simulink model "AAIR4"  (R2020a)
settings: Solver=FixedStepAuto  StartTime=0.0  StopTime=10.0  FixedStep=1e-3  RelTol=1e-3  EnableMultiTasking=on
undefined symbols (not defined in the file): D0, D10, D11, D13, D2, D4, D5, D6, D8, PTA0, PTA2, PTB23, PTB9, PTC16, PTC2, PTD0, PTD1, PTD2
libraries: frdmk64flib x15, dspstat3 x1
settings Model: ExtModeTrigDuration=5  Creator=guga  LastModifiedBy=guga
settings OptimizationCC: EnhancedBackFolding=on  PassReuseOutputArgsAs=Individual arguments  ZeroExternalMemoryAtStartup=off  ZeroInternalMemoryAtStartup=off  MaxStackSize=64  OptimizeBlockOrder=speed  DifferentSizesBufferReuse=on  OptimizationCustomize=off  EfficientTunableParamExpr=on
settings DebuggingCC: ParameterTunabilityLossMsg=error
settings HardwareCC: ProdBitPerPointer=32  ProdBitPerSizeT=32  ProdBitPerPtrDiffT=32  ProdLargestAtomicInteger=Long  ProdLargestAtomicFloat=Double  ProdWordSize=32  ProdHWDeviceType=ARM Compatible->ARM Cortex
settings SFSimCC: MATLABDynamicMemAlloc=off
settings RTWCC: SystemTargetFile=ert.tlc  HardwareBoard=NXP FRDM-K64F  TemplateMakefile=ert_default_tmf  Toolchain=GNU Tools for ARM Embedded Processors
settings CodeAppCC: ForceParamTrailComments=on  IgnoreCustomStorageClasses=off  OperatorAnnotations=on  SimulinkDataObjDesc=on  SFDataObjDesc=on  InsertBlockDesc=on

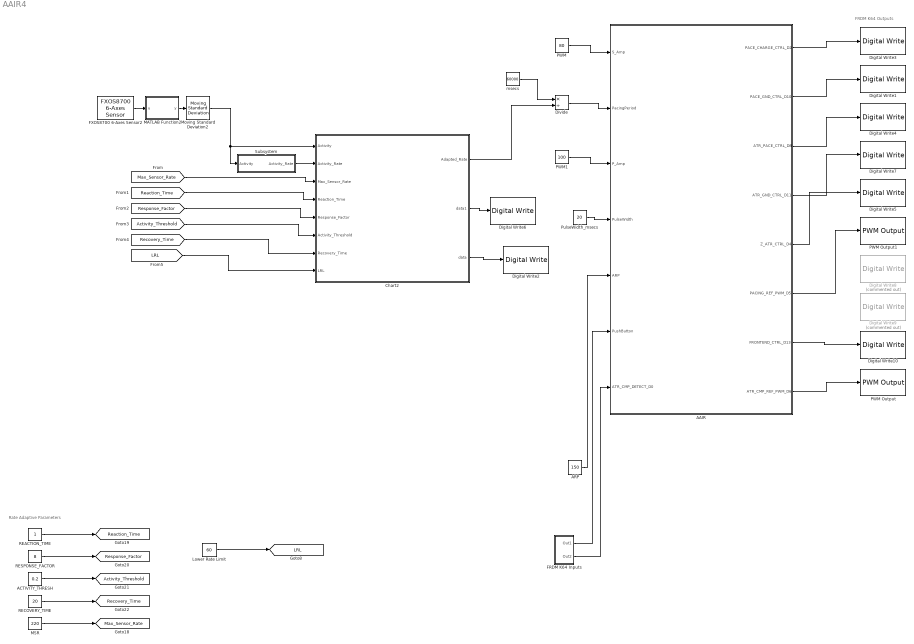
== system AAIR4 ==
  note: FRDM K64 Outputs
  note: Rate Adaptive Parameters
  AAIR : Stateflow chart  TreatAsAtomicUnit=on
  ACTIVITY_THRESH : Constant  Value=0.2  OutDataTypeStr=double
  ARP : Constant  Value=150
  Chart2 : Stateflow chart  TreatAsAtomicUnit=on
  Digital Write1 : frdmk64flib/Digital Write  Whichpin=PTD0 (D10)
  Digital Write10 : frdmk64flib/Digital Write  Whichpin=PTD1 (D13)
  Digital Write2 : frdmk64flib/Digital Write  Whichpin=RED_LED
  Digital Write3 : frdmk64flib/Digital Write  Whichpin=PTB9 (D2)
  Digital Write4 : frdmk64flib/Digital Write  Whichpin=PTA0 (D8)
  Digital Write5 : frdmk64flib/Digital Write  Whichpin=PTB23 (D4)
  Digital Write6 : frdmk64flib/Digital Write  Whichpin=GREEN_LED
  Digital Write7 : frdmk64flib/Digital Write  Whichpin=PTD2 (D11)
  Digital Write8 : frdmk64flib/Digital Write  Commented=on  Whichpin=RED_LED
  Digital Write9 : frdmk64flib/Digital Write  Commented=on  Whichpin=GREEN_LED
  Divide : Product  Inputs=*/
  FRDM K64 Inputs : Subsystem
  FXOS8700 6-Axes Sensor2 : frdmk64flib/FXOS8700 6-Axes Sensor  Activesensor=Accelerometer only  ODR=100Hz  HybridODR=400Hz  Accelfullrange=-4g to +4g  SampleTime=1/100
  Lower Rate Limit : Constant  Value=60  OutDataTypeStr=uint16
  MATLAB Function2 : MATLAB Function  TreatAsAtomicUnit=on
  MSR : Constant  Value=220  OutDataTypeStr=uint16
  Moving Standard Deviation2 : dspstat3/Moving Standard Deviation  Method=Sliding window  ForgettingFactorPort=off  SpecifyWindowLength=on  WindowLength=100  ForgettingFactor=0.9  SimulateUsing=Code generation
      settings: SourceProductBaseCode=DS
  PWM : Constant  Value=80
  PWM Output : frdmk64flib/PWM Output  Whichpin=PTC2 (D6)  InitialFrequency=2000  InitialDutyCycle=0
  PWM Output1 : frdmk64flib/PWM Output  Whichpin=PTA2 (D5)  InitialFrequency=2000  InitialDutyCycle=0
  PWM1 : Constant  Value=100
  PulseWidth_msecs : Constant  Value=20
  "REACTION_TIME " : Constant  OutDataTypeStr=uint16
  RECOVERY_TIME : Constant  Value=20  OutDataTypeStr=uint16
  RESPONSE_FACTOR : Constant  Value=8  OutDataTypeStr=double  LockScale=on
  Subsystem : Subsystem
  msecs : Constant  Value=60000
  tag scope: Activity_Threshold=global, LRL=global, Max_Sensor_Rate=global, Reaction_Time=global, Recovery_Time=global, Response_Factor=global
  wires:
  PulseWidth_msecs/1 -> AAIR/4(PulseWidth)
  PWM1/1 -> AAIR/3(P_Amp)
  Divide/1 -> AAIR/2(PacingPeriod)
  PWM/1 -> AAIR/1(S_Amp)
  Chart2/1(Adapted_Rate) -> Divide/2
  msecs/1 -> Divide/1
  FRDM K64 Inputs/1(Out1) -> AAIR/6(PushButton)
  FRDM K64 Inputs/2(Out2) -> AAIR/7(ATR_CMP_DETECT_D0)
  ARP/1 -> AAIR/5(ARP)
  [Recovery_Time] -> Chart2/7(Recovery_Time)
  [Response_Factor] -> Chart2/5(Response_Factor)
  FXOS8700 6-Axes Sensor2/1 -> MATLAB Function2/1(u)
  [Reaction_Time] -> Chart2/4(Reaction_Time)
  [Max_Sensor_Rate] -> Chart2/3(Max_Sensor_Rate)
  Moving Standard Deviation2/1 -> Chart2/1(Activity), Subsystem/1(Activity)
  MATLAB Function2/1(y) -> Moving Standard Deviation2/1
  Subsystem/1(Activity_Rate) -> Chart2/2(Activity_Rate)
  [LRL] -> Chart2/8(LRL)
  [Activity_Threshold] -> Chart2/6(Activity_Threshold)
  "REACTION_TIME "/1 -> [Reaction_Time]
  RESPONSE_FACTOR/1 -> [Response_Factor]
  ACTIVITY_THRESH/1 -> [Activity_Threshold]
  RECOVERY_TIME/1 -> [Recovery_Time]
  MSR/1 -> [Max_Sensor_Rate]
  Lower Rate Limit/1 -> [LRL]
  AAIR/6(PACING_REF_PWM_D5) -> PWM Output1/1
  AAIR/2(PACE_GND_CTRL_D10) -> Digital Write1/1
  AAIR/4(ATR_GND_CTRL_D11) -> Digital Write7/1
  AAIR/1(PACE_CHARGE_CTRL_D2) -> Digital Write3/1
  AAIR/5(Z_ATR_CTRL_D4) -> Digital Write5/1
  AAIR/3(ATR_PACE_CTRL_D8) -> Digital Write4/1
  AAIR/7(FRONTEND_CTRL_D13) -> Digital Write10/1
  AAIR/8(ATR_CMP_REF_PWM_D6) -> PWM Output/1
  Chart2/3(data) -> Digital Write2/1
  Chart2/2(data1) -> Digital Write6/1

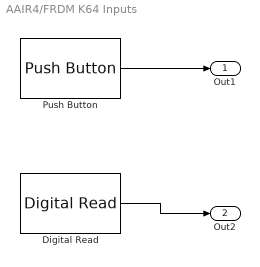
== system AAIR4/FRDM K64 Inputs ==
  Digital Read : frdmk64flib/Digital Read  Whichpin=PTC16 (D0)  SampleTime=-1
  Push Button : frdmk64flib/Push Button  Whichswitch=SW2  SampleTime1=-1
  Out1 : Outport
  Out2 : Outport  Port=2
  wires:
  Digital Read/1 -> Out2/1
  Push Button/1 -> Out1/1

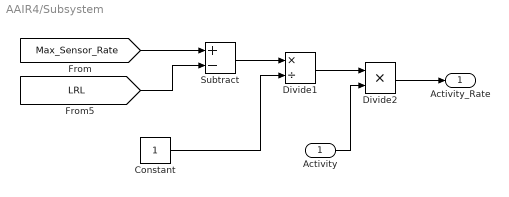
== system AAIR4/Subsystem ==
  Activity : Inport
  Constant : Constant
  Divide1 : Product  Inputs=*/
  Divide2 : Product  Inputs=**  OutDataTypeStr=uint16
  Subtract : Sum  Inputs=+-
  Activity_Rate : Outport  VectorParamsAs1DForOutWhenUnconnected=off
  wires:
  [Max_Sensor_Rate] -> Subtract/1
  [LRL] -> Subtract/2
  Subtract/1 -> Divide1/1
  Divide1/1 -> Divide2/1
  Activity/1 -> Divide2/2
  Divide2/1 -> Activity_Rate/1
  Constant/1 -> Divide1/2

== stateflow chart AAIR4/Chart2 ==
  state Update_Rate [commented out]
  state Activity_Rate
    entry:
    data = true;
    exit:
    data = false;
  state Up
    entry:
    Time = 0;
    data1 = true;
    during:
    Adapted_Rate = Response_Factor*(Time/Reaction_Time)/(1+(Time/Reaction_Time)*(Response_Factor-1))*Activity_Rate + LRL;
    Time = Time + 1/1000;
    exit:
    Time = 0;
    data1 = false;
  state Max
    entry:
    Adapted_Rate = Max_Sensor_Rate;
  state Down
    entry:
    Time = 0;
    Rate_Diff = Adapted_Rate - LRL;
    during:
    Adapted_Rate = Adapted_Rate - (Rate_Diff/Recovery_Time)*Time;
    Time = Time + 1/1000;
    exit:
    Time = 0;
  state Start
    entry:
    Adapted_Rate = LRL;
  state Min
  Up -> Update_Rate [commented out] : [after(10, msec)]
  Update_Rate -> Up [commented out] : [after(10, msec)]
  Up -> Activity_Rate [order 2] : [Adapted_Rate>=Activity_Rate+LRL]{Time = 0}
  Up -> Up [order 3] : [Time >= Reaction_Time]{Time = 0}
  Activity_Rate -> Down [order 2] : [Activity < Activity_Threshold]
  Activity_Rate -> Up [order 1] : [Activity >= Activity_Threshold]{Time = 0}
  Up -> Max [order 1] : [Adapted_Rate >= Max_Sensor_Rate]{Time = 0}
  Min -> Up : [Activity >= Activity_Threshold]{Time = 0}
  Max -> Down : [Activity < Activity_Threshold]
  Up -> Down [order 4] : [Activity < Activity_Threshold]{Time = 0}
  Down -> Up [order 1] : [Activity >= Activity_Threshold]{Time = 0}
  (default) -> Start
  Start -> Down
  Down -> Min [order 2] : [Adapted_Rate == LRL]
  Down -> Down [order 3] : [Time >= Recovery_Time]{Time = 0}
  data: Activity input double; Activity_Rate input; Adapted_Rate output uint16; data1 output; Max_Sensor_Rate input uint16; Reaction_Time input uint16; Response_Factor input double; Activity_Threshold input double; Recovery_Time input uint16; LRL input uint16; Rate_Diff local uint16; Time local double; data output

== matlab function AAIR4/MATLAB Function2 ==
  data: u input; y output
function y = fcn(u)
y = sqrt(u(1)^2+u(2)^2+u(3)^2);

== stateflow chart AAIR4/AAIR ==
  state Pacing
    entry:
    PACING_REF_PWM_D5 = P_Amp;
    PACE_CHARGE_CTRL_D2=0;
    ATR_PACE_CTRL_D8= 1;
    ATR_GND_CTRL_D11= 0;
    PACE_GND_CTRL_D10=1;
    Z_ATR_CTRL_D4=0;
    %LED_STATE_RED=0;
    %LED_STATE_GREEN=0;
  state Charging_and_Sensing
    entry:
    PACING_REF_PWM_D5 = P_Amp;
    PACE_CHARGE_CTRL_D2=1;
    ATR_PACE_CTRL_D8= 0;
    ATR_GND_CTRL_D11= 1;
    PACE_GND_CTRL_D10=0;
    Z_ATR_CTRL_D4=0;
    %LED_STATE_RED=0;
    %LED_STATE_GREEN=0;
    FRONTEND_CTRL_D13 = 1;
    ATR_CMP_REF_PWM_D6 = S_Amp;
  (default) -> Charging_and_Sensing
  Pacing -> Charging_and_Sensing : after(PulseWidth,msec)
  Charging_and_Sensing -> (junction 85) : after(ARP-PulseWidth, msec)
  (junction 85) -> Pacing [order 2] : after(PacingPeriod-ARP,msec)[ATR_CMP_DETECT_D0 == 0 & PushButton == false]
  (junction 85) -> Charging_and_Sensing [order 1] : [ATR_CMP_DETECT_D0 == 1 | PushButton == true]
  data: S_Amp input; PacingPeriod input; A_Atrium local; V_Ventricle local; I_Inhibited local; O_None local; VENT_CMP_DETECT_D1 local; VENT_CMP_REF_PWM_D3 local; Z_VENT_CTRL_D7 local; VENT_PACE_CTRL_D9 local; VENT_GND_CTRL_D12 local; GND local; VENT_RECT_SIGNAL_A4_SDA local; ATR_RECT_SIGNAL_A3 local; Z_SIGNAL_A2 local; VENT_SIGNAL_A1 local; ATR_SIGNAL_A0 local; PACE_CHARGE_CTRL_D2 output; PACE_GND_CTRL_D10 output; ATR_PACE_CTRL_D8 output; ATR_GND_CTRL_D11 output; Z_ATR_CTRL_D4 output; PACING_REF_PWM_D5 output; P_Amp input; PulseWidth input; ARP input; PushButton input; FRONTEND_CTRL_D13 output; ATR_CMP_DETECT_D0 input; ATR_CMP_REF_PWM_D6 output
